simulink model "ev-obc-active-power-decoupling-model"  (R2025a)
settings: Solver=FixedStepAuto  StartTime=0.0  StopTime=1  FixedStep=1e-6  RelTol=1e-3
undefined symbols (not defined in the file): C_aux, k_current, k_power_alpha, k_power_beta, k_voltage, L_g, T_sw, Vbatt, w0
libraries: nesl_utility x12, fl_lib x11, ee_lib x4, spsAlphaBetaZerotodq0Lib x3, eeGeneralControl x2, slpidlib x2, spsdq0toAlphaBetaZeroLib x2
settings Model: Creator=AnasJ  LastModifiedBy=MEET

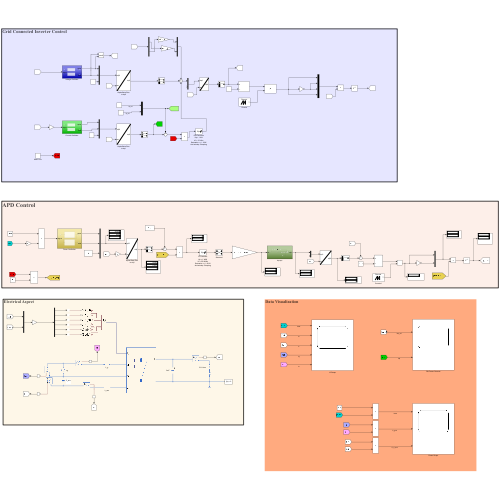
[thumbnail: Simulink's stored preview of the top-level diagram]
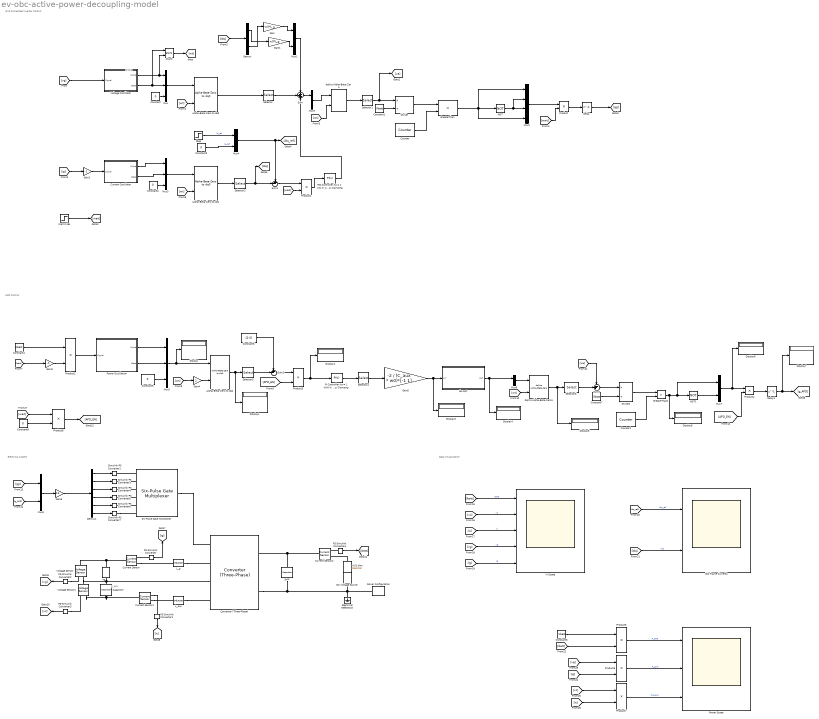
== system ev-obc-active-power-decoupling-model ==
  note: Data Visualization
  note: Electrical Aspect
  note: C_aux
  note: APD Control
  note: Grid Connected Inverter Control
  note: Alpha
  0.01 ohm : fl_lib/Electrical/Electrical Elements/Resistor  R=0.2 Ohm  i_specify=off  i_priority=None  i=0 A  i_nominal_specify=off  i_nominal_value=1  i_nominal_unit=A  v_specify=off  v_priority=None  v=0 V  v_nominal_specify=off  v_nominal_value=1  v_nominal_unit=V
  3mF : fl_lib/Electrical/Electrical Elements/Capacitor  c=3e-3 F  r=1e-6 Ohm  g=0 1/Ohm  i_specify=off  i_priority=None  i=0 A  i_nominal_specify=off  i_nominal_value=1  i_nominal_unit=A  v_specify=on  v_priority=High  v=400 V  v_nominal_specify=off  v_nominal_value=1  v_nominal_unit=V  vc_specify=off  vc_priority=High  vc=0 V  vc_nominal_specify=off  vc_nominal_value=1  vc_nominal_unit=V
  Alpha-Beta-Zero to dq0 : spsAlphaBetaZerotodq0Lib/Alpha-Beta-Zero to dq0  Alignment=90 degrees behind phase A axis
  Alpha-Beta-Zero to dq1 : spsAlphaBetaZerotodq0Lib/Alpha-Beta-Zero to dq0  Alignment=90 degrees behind phase A axis
  Alpha-Beta-Zero to dq2 : spsAlphaBetaZerotodq0Lib/Alpha-Beta-Zero to dq0  Alignment=90 degrees behind phase A axis
  Atan2 : Trigonometry  Operator=atan2
  Capacitor : fl_lib/Electrical/Electrical Elements/Capacitor  c=460 uF  r=1e-6 Ohm  g=0 1/Ohm  i_specify=off  i_priority=None  i=0 A  i_nominal_specify=off  i_nominal_value=1  i_nominal_unit=A  v_specify=off  v_priority=High  v=0 V  v_nominal_specify=off  v_nominal_value=1  v_nominal_unit=V  vc_specify=off  vc_priority=High  vc=0 V  vc_nominal_specify=off  vc_nominal_value=1  vc_nominal_unit=V
  Constant{,2..3,5,9} (5 alike) : Constant  Value=0
  Constant{1,4,7..8} (4 alike) : Constant  Value=Vbatt
  Constant6 : Constant  Value=[0 0]
  Converter (Three-Phase) : ee_lib/Semiconductors & Converters/Converters/Converter (Three-Phase)  port_option=ee.enum.threePhasePort.expanded  fidelity_option=ee.enum.converters.fidelity.detailed  device_type=ee.enum.converters.switchingdevice.ideal  showThermalPort=false  K=0  Vth=6 V  Vgt=1 V  Vgt_off=-1 V  Ih=1 A  Vf=0.8 V  Ron=0.001 Ohm  Rds=0.001 Ohm  Goff=1e-6 1/Ohm  Eon_scalar=22.86e-3 J  Eoff_scalar=17.14e-3 J  Eoff_natural_commutation=10e-3 J  Voff=300 V  Iout_scalar=600 A  onCurrentMeasDelay=0 s  useCurrentFromPreviousCycle=false  useVoltageFromPreviousCycle=false  diode_param=ee.enum.converters.protectiondiode.nodynamics  diode_Vf=0.8 V  diode_Ron=0.001 Ohm  diode_Goff=1e-5 1/Ohm  diode_C=50 nF  diode_iRM=-235 A  diode_iF=300 A  diode_idot=-50 A/us  diode_trr_param=ee.enum.converters.diodetrr.trr_factor  diode_trr_factor=3  diode_trr=15 us  diode_Qrr=1500 s*uA  diode_rec_loss_model=ee.enum.diode.reverseRecoveryModel.fixed  diode_ErecVal=0 J  diode_scaleWithIandV=false  diode_ErecMat=zeros(2, 3) J  diode_TjrecVec=[298.15, 398.15] K  diode_IfrecVec=[.1, 1, 10] A  diode_IrecVal=10 A  diode_VrecVal=10 V  diode_tFilter=1 / 1000 / 100 s  thermal_network_parameterization=ee.enum.thermalNetworkTopology.external  Rth=[.08, .5] K/W  Rth_Cauer=[.08, .1, .5] K/W  Rth_Foster=[.08, .14, .22, .16] K/W  thermal_mass_parameterization=ee.enum.thermalNetwork.timeconstant  thermal_mass=[.01, .5] J/K  thermal_mass_Cauer=[.01, .1, .5] J/K  thermal_mass_Foster=[.001, .005, .05, .5] J/K  thermal_time_constant=[.001, .2] s  thermal_time_constant_Cauer=[.001, .1, .2] s  thermal_time_constant_Foster=[7e-05, .0007, .01, .08] s  thermal_mass_initial_temperatures=[25, 25] degC  thermal_mass_initial_temperatures_Cauer=[25, 25, 25] degC  junction_thermal_mass=0.01 J/K  Tvec_initial_Foster=[25, 25, 25, 25] degC  snubber_type=ee.enum.converters.snubber.include  Cs=1e-7 F  Rs=0.1 Ohm  Vce_loss=[0, 150, 300] V
      settings: InternalSimscapePortConfiguration="{\"Bottom\":[],\"Left\":[{\"id\":\"G\",\"label\":\"G\",\"type\":\"foundation.electrical.twelve_phase\"},{\"id\":\"a\",\"label\":\"a\",\"type\":\"foundation.electrical.electrical\"},{\"id\":\"b\",\"label\":\"b\",\"type\":\"foundation.electrical.electrical\"},{\"id\":\"c\",\"label\":\"c\",\"type\":\"foundation.electrical.electrical\"}],\"Right\":[{\"id\":\"p\",\"label\":\"+\",\"type\":\"foundation.electrical.electrical\"},{\"id\":\"n\",\"label\":\"-\",\"type\":\"foundation.electrical.electrical\"}],\"Top\":[]}"
  Counter : eeGeneralControl/Counter  CarrCount=Up  Range=[0 1]  Tper=0.15  Tdelay=0  Ts=T_sw
      settings: LibrarySourceBlock=ee_sl_lib/General Control/Counter
  Counter1 : eeGeneralControl/Counter  CarrCount=Up  Range=[0 1]  Tper=0.15  Tdelay=0  Ts=T_sw
      settings: LibrarySourceBlock=ee_sl_lib/General Control/Counter
  Current Oscillator : Subsystem
  Current Sensor : fl_lib/Electrical/Electrical Sensors/Current Sensor
  Current Sensor1 : fl_lib/Electrical/Electrical Sensors/Current Sensor
  Current Sensor2 : fl_lib/Electrical/Electrical Sensors/Current Sensor
  DC Voltage Source : fl_lib/Electrical/Electrical Sources/DC Voltage Source  v0=400 V
  DQ Frame Currents : Scope  NumInputPorts=2
      settings: ActiveDisplayYMinimum=-56.25  ActiveDisplayYMaximum=6.2499999999999982
  Delay : Delay  DelayLength=1  InputProcessing=Columns as channels (frame based)
  Delay1 : Delay  DelayLength=1  InputProcessing=Columns as channels (frame based)
  Demux : Demux  Outputs=2
  Demux1 : Demux  Outputs=6
  Display{,1..8} (9 alike) : Display
  Divide : Product  Inputs=*/
  Divide1 : Product  Inputs=*/
  Electrical Reference : fl_lib/Electrical/Electrical Elements/Electrical Reference
  Gain : Gain  Gain=-w0*L_g
  Gain1 : Gain  Gain=w0*L_g
  Gain2 : Gain  Gain=-1
  Gain3 : Gain  Gain=-1
  Gain4 : Gain  Gain=2
  Gain5 : Gain  Gain=-2 / (C_aux * w0)*[-1 1]
  Gain6 : Gain  Gain=12
  GreaterThan : RelationalOperator  Operator=>  OutDataTypeStr=boolean  RndMeth=Simplest  InputSameDT=off
  GreaterThan1 : RelationalOperator  Operator=>  OutDataTypeStr=boolean  RndMeth=Simplest  InputSameDT=off
  L_aux : ee_lib/Passive/Inductor  l=55e-6 H  enable_L_tol=ee.enum.toleranceApplication.none  L_tol=20  tol_distribution=ee.enum.toleranceDistribution.uniform  nSigma=4  r=0.2 Ohm  g=1e-9 1/Ohm  enable_operating_limits=ee.enum.enable.no  operating_limit_action=ee.enum.passive.reportOpLim.warn  max_working_current=1 A  power_rating=1 W  i_L_specify=off  i_L_priority=High  i_L=0 A  i_L_nominal_specify=off  i_L_nominal_value=1  i_L_nominal_unit=A
  L_g : ee_lib/Passive/Inductor  l=16.35 mH  enable_L_tol=ee.enum.toleranceApplication.none  L_tol=20  tol_distribution=ee.enum.toleranceDistribution.uniform  nSigma=4  r=0.2 Ohm  g=1e-9 1/Ohm  enable_operating_limits=ee.enum.enable.no  operating_limit_action=ee.enum.passive.reportOpLim.warn  max_working_current=1 A  power_rating=1 W  i_L_specify=off  i_L_priority=High  i_L=0 A  i_L_nominal_specify=off  i_L_nominal_value=1  i_L_nominal_unit=A
  Mux : Mux  Inputs=3
  Mux{1,4,6..9} (6 alike) : Mux  Inputs=2
  Mux2 : Mux
  Mux3 : Mux  Inputs=3
  Mux5 : Mux  Inputs=3
  NOT : Logic  Operator=NOT  IconShape=distinctive  AllPortsSameDT=off  OutDataTypeStr=boolean
  NOT1 : Logic  Operator=NOT  IconShape=distinctive  AllPortsSameDT=off  OutDataTypeStr=boolean
  PI Controller Kp = 1 W/W Ki = 25 W/Ws Saturation = +/- 5e3V Anti-windup: Clamping : slpidlib/PID Controller  Controller=PI  Form=Parallel  TimeDomain=Continuous-time  UseExternalTs=off  SampleTime=-1  IntegratorMethod=Forward Euler  FilterMethod=Forward Euler  ControllerParametersSource=internal  P=1  I=25  UseKiTs=off  D=0  UseExternalDerivativeSource=off  N=100  UseFilter=on  TunerSelectOption=Transfer Function Based (PID Tuner App)  InitialConditionSource=internal  InitialConditionForIntegrator=0  InitialConditionForFilter=0  DifferentiatorICPrevScaledInput=0  ExternalReset=none  TrackingMode=off  Kt=1  LimitOutput=on  SatLimitsSource=internal  UpperSaturationLimit=5e3  LowerSaturationLimit=-5e3  LinearizeAsGain=on  AntiWindupMode=none  Kb=1  LimitIntegrator=off  UpperIntegratorSaturationLimit=inf  LowerIntegratorSaturationLimit=-inf  POutMin=[]  POutMax=[]  IOutMin=[]  IOutMax=[]  DOutMin=[]  DOutMax=[]  NOutMin=[]  NOutMax=[]  SumOutMin=[]  SumOutMax=[]  SaturationOutMin=[]  SaturationOutMax=[]  PParamMin=[]  PParamMax=[]  IParamMin=[]  IParamMax=[]  DParamMin=[]  DParamMax=[]  NParamMin=[]  NParamMax=[]  KbParamMin=[]  KbParamMax=[]  KtParamMin=[]  KtParamMax=[]  KbOutMin=[]  KbOutMax=[]  KtOutMin=[]  KtOutMax=[]  IntegratorOutMin=[]  IntegratorOutMax=[]  FilterOutMin=[]  FilterOutMax=[]  SumI1OutMin=[]  SumI1OutMax=[]  SumI2OutMin=[]  SumI2OutMax=[]  SumI3OutMin=[]  SumI3OutMax=[]  SumI4OutMin=[]  SumI4OutMax=[]  SumDOutMin=[]  SumDOutMax=[]  DifferentiatorOutMin=[]  DifferentiatorOutMax=[]  FilterDiffOutCoefMin=[]  FilterDiffOutCoefMax=[]  ReciprocalOutMin=[]  ReciprocalOutMax=[]  SumDenOutMin=[]  SumDenOutMax=[]  SumNumOutMin=[]  SumNumOutMax=[]  DivideOutMin=[]  DivideOutMax=[]  UdiffTsProdOutMin=[]  UdiffTsProdOutMax=[]  NTsProdOutMin=[]  NTsProdOutMax=[]  UintegralTsProdOutMin=[]  UintegralTsProdOutMax=[]  UngainTsProdOutMin=[]  UngainTsProdOutMax=[]  ClampingZeroOutDataTypeStr=Inherit: Inherit via back propagation  ClampingZeroOutMin=[]  ClampingZeroOutMax=[]  FilterDenConstantOutDataTypeStr=Inherit: Inherit via back propagation  FilterDenConstantOutMin=[]  FilterDenConstantOutMax=[]  PCopyOutDataTypeStr=Inherit: Inherit via back propagation  PCopyOutMin=[]  PCopyOutMax=[]  NCopyOutDataTypeStr=Inherit: Inherit via back propagation  NCopyOutMin=[]  NCopyOutMax=[]  IntegratorContinuousStateAttributes=''  IntegratorStateMustResolveToSignalObject=off  IntegratorRTWStateStorageClass=Auto  FilterContinuousStateAttributes=''  FilterStateMustResolveToSignalObject=off  FilterRTWStateStorageClass=Auto  ParallelPVariant=InternalParameters  IdealPVariant=Disabled  IVariant=InternalParameters  DVariant=Disabled  IntegratorVariant=Continuous  SatVariant=Enabled  AWVariant=Passthrough  PCopyVariant=Disabled  TRVariant=Disabled  FdbkBlocksVariant=Forward  IdealPFdbkVariant=Disabled  SatFdbkVariant=Disabled  DerivativeFilterVariant=Disabled  NVariant=Disabled  NCopyVariant=Disabled_SignalSpec  FilterICVariant=Disabled  IntegratorICVariant=InternalICs  ExternalResetVariant=Disabled  TRSumVariant=Passthrough  SumFdbkVariant=Disabled  SumVariant=Sum_PI  TsampFilterVariant=InternalTs  TsampNgainVariant=Passthrough  TsampIntegralVariant=Disabled_SignalSpec  ExternalSaturationOutDataTypeStr=Inherit: Same as second input  DerivativeSourceVariant=Disabled  PreIntVariant=InternalPreInt
  PID Controller Kp = 1 V/A Ki = 10 V/As Saturation = +/- 100V Anti-windup: Clamping : slpidlib/PID Controller  Controller=PI  Form=Parallel  TimeDomain=Continuous-time  UseExternalTs=off  SampleTime=-1  IntegratorMethod=Forward Euler  FilterMethod=Forward Euler  ControllerParametersSource=internal  P=5  I=50  UseKiTs=off  D=0  UseExternalDerivativeSource=off  N=100  UseFilter=on  TunerSelectOption=Transfer Function Based (PID Tuner App)  InitialConditionSource=internal  InitialConditionForIntegrator=0  InitialConditionForFilter=0  DifferentiatorICPrevScaledInput=0  ExternalReset=none  TrackingMode=off  Kt=1  LimitOutput=on  SatLimitsSource=internal  UpperSaturationLimit=100  LowerSaturationLimit=-100  LinearizeAsGain=on  AntiWindupMode=clamping  Kb=1  LimitIntegrator=off  UpperIntegratorSaturationLimit=inf  LowerIntegratorSaturationLimit=-inf  POutMin=[]  POutMax=[]  IOutMin=[]  IOutMax=[]  DOutMin=[]  DOutMax=[]  NOutMin=[]  NOutMax=[]  SumOutMin=[]  SumOutMax=[]  SaturationOutMin=[]  SaturationOutMax=[]  PParamMin=[]  PParamMax=[]  IParamMin=[]  IParamMax=[]  DParamMin=[]  DParamMax=[]  NParamMin=[]  NParamMax=[]  KbParamMin=[]  KbParamMax=[]  KtParamMin=[]  KtParamMax=[]  KbOutMin=[]  KbOutMax=[]  KtOutMin=[]  KtOutMax=[]  IntegratorOutMin=[]  IntegratorOutMax=[]  FilterOutMin=[]  FilterOutMax=[]  SumI1OutMin=[]  SumI1OutMax=[]  SumI2OutMin=[]  SumI2OutMax=[]  SumI3OutMin=[]  SumI3OutMax=[]  SumI4OutMin=[]  SumI4OutMax=[]  SumDOutMin=[]  SumDOutMax=[]  DifferentiatorOutMin=[]  DifferentiatorOutMax=[]  FilterDiffOutCoefMin=[]  FilterDiffOutCoefMax=[]  ReciprocalOutMin=[]  ReciprocalOutMax=[]  SumDenOutMin=[]  SumDenOutMax=[]  SumNumOutMin=[]  SumNumOutMax=[]  DivideOutMin=[]  DivideOutMax=[]  UdiffTsProdOutMin=[]  UdiffTsProdOutMax=[]  NTsProdOutMin=[]  NTsProdOutMax=[]  UintegralTsProdOutMin=[]  UintegralTsProdOutMax=[]  UngainTsProdOutMin=[]  UngainTsProdOutMax=[]  ClampingZeroOutDataTypeStr=Inherit: Inherit via back propagation  ClampingZeroOutMin=[]  ClampingZeroOutMax=[]  FilterDenConstantOutDataTypeStr=Inherit: Inherit via back propagation  FilterDenConstantOutMin=[]  FilterDenConstantOutMax=[]  PCopyOutDataTypeStr=Inherit: Inherit via back propagation  PCopyOutMin=[]  PCopyOutMax=[]  NCopyOutDataTypeStr=Inherit: Inherit via back propagation  NCopyOutMin=[]  NCopyOutMax=[]  IntegratorContinuousStateAttributes=''  IntegratorStateMustResolveToSignalObject=off  IntegratorRTWStateStorageClass=Auto  FilterContinuousStateAttributes=''  FilterStateMustResolveToSignalObject=off  FilterRTWStateStorageClass=Auto  ParallelPVariant=InternalParameters  IdealPVariant=Disabled  IVariant=InternalParameters  DVariant=Disabled  IntegratorVariant=Continuous  SatVariant=Enabled  AWVariant=ContClampingParallel  PCopyVariant=Disabled  TRVariant=Disabled  FdbkBlocksVariant=Forward  IdealPFdbkVariant=Disabled  SatFdbkVariant=Disabled  DerivativeFilterVariant=Disabled  NVariant=Disabled  NCopyVariant=Disabled_SignalSpec  FilterICVariant=Disabled  IntegratorICVariant=InternalICs  ExternalResetVariant=Disabled  TRSumVariant=Passthrough  SumFdbkVariant=Disabled  SumVariant=Sum_PI  TsampFilterVariant=InternalTs  TsampNgainVariant=Passthrough  TsampIntegralVariant=Disabled_SignalSpec  ExternalSaturationOutDataTypeStr=Inherit: Same as second input  DerivativeSourceVariant=Disabled  PreIntVariant=InternalPreInt
  PS-Simulink Converter{,1..4} (5 alike) : nesl_utility/PS-Simulink Converter  PhysicalDomain=network_engine_domain  SubClassName=ps_output  LeftPortType=input  RightPortType=output  PseudoPeriodic=off  Frequencies=[]  VectorFormat=inherit  Unit=inherit  AffineConversion=off
  Power Oscillation : Subsystem
  Power Scope : Scope  NumInputPorts=3
      settings: ActiveDisplayYMinimum=-891089.21436589747  ActiveDisplayYMaximum=99010.920853026575  DataLoggingVariableName=ScopeData2
  Product{,1..8} (9 alike) : Product
  Selector : Selector  InputPortWidth=3  IndexOptions=Index vector (dialog)  Indices=[1 2]  OutputSizes=1
  Selector1 : Selector  InputPortWidth=3  IndexOptions=Index vector (dialog)  Indices=[1]  OutputSizes=1
  Selector2 : Selector  InputPortWidth=3  IndexOptions=Index vector (dialog)  Indices=[1 2]  OutputSizes=1
  Selector3 : Selector  InputPortWidth=3  IndexOptions=Index vector (dialog)  Indices=[1 2]  OutputSizes=1
  Selector4 : Selector  InputPortWidth=2  IndexOptions=Index vector (dialog)  Indices=[2 1]  OutputSizes=1
  Selector5 : Selector  InputPortWidth=3  IndexOptions=Index vector (dialog)  Indices=[1]  OutputSizes=1
  Simulink-PS Converter{1,3..7} (6 alike) : nesl_utility/Simulink-PS Converter  PhysicalDomain=network_engine_domain  SubClassName=ps_input  LeftPortType=input  RightPortType=output  PseudoPeriodic=off  Frequencies=[]  NoiseDistribution=none  NoiseParameters=[]  Unit=1  AffineConversion=off  FilteringAndDerivatives=provide  SimscapeFilterOrder=1  InputFilterTimeConstant=0.001  UdotUserProvided=0
  Six-Pulse Gate Multiplexer : ee_lib/Semiconductors & Converters/Converters/Six-Pulse Gate Multiplexer  port_option=ee.enum.controlport.ps
  Solver Configuration : nesl_utility/Solver Configuration  PhysicalDomain=network_engine_domain  SubClassName=solver  LeftPortType=input  RightPortType=generic  Tones=[]  Harmonics=[]  SimulateNoise=off  Profile=off  UseLocalSampling=off  EnableSwitchedLinearOptims=on  FrequencyDomain=off  UseCCode=off  RelTol=0.001  AbsTol=0.001  MinStep=1e-09  ToWorkspace=off  RevertToSquareIcSolve=off  NumHomotopyIterations=100  PhasorMode=off  PhasorModeNumHarmonics=1  ConsistencySolver=NEWTON_XTOL_AFTER_FTOL  IndexReductionMethod=DerivativeReplacement  DoDC=off  ResidualTolerance=1e-09  ConsistencyTolSource=GLOBAL  ConsistencyAbsTol=0.001  ConsistencyRelTol=0.001  ConsistencyTolFactor=0.001  UseLocalSolver=on  LocalSolverChoice=NE_TRAPEZOIDAL_ADVANCER  ResolveIndetEquations=on  FunctionEvalNumThread=1  LocalSolverSampleTime=1e-6  DoFixedCost=off  MaxNonlinIter=3  MaxModeIter=2  ComputeImpulses=off  ImpulseIterations=2  LinearAlgebra=auto  LinearAlgebraNumThread=0  EquationFormulation=NE_TIME_EF  DelaysMemoryBudget=1024  AutomaticFiltering=on  FilteringTimeConstant=0.001  PartitionStorageMethod=AS_NEEDED  PartitionMemoryBudget=1024  PartitionMethod=ROBUST  MultibodyUseLocalSolver=off  MultibodyLocalSolverChoice=ODE1  MultibodyLocalSolverSampleTime=0.001
  Step : Step  Time=0.2  After=-50  SampleTime=0
  Sum : Sum  Inputs=+++
  Sum1 : Sum  Inputs=+-|
  Sum2 : Sum  Inputs=+-|
  Sum3 : Sum  Inputs=-+|
  VI Scope : Scope  NumInputPorts=5
      settings: ActiveDisplayYMinimum=-2227.7230359147438  ActiveDisplayYMaximum=247.52730213256646
  Voltage Oscillator : Subsystem
  Voltage Sensor : fl_lib/Electrical/Electrical Sensors/Voltage Sensor
  Voltage Sensor1 : fl_lib/Electrical/Electrical Sensors/Voltage Sensor
  Wait 0.15s : Step  Time=0.15  SampleTime=0
  dq-sqrt : Subsystem
  dq0 to Alpha-Beta-Zero : spsdq0toAlphaBetaZeroLib/dq0 to Alpha-Beta-Zero  Alignment=90 degrees behind phase A axis
  dq0 to Alpha-Beta-Zero1 : spsdq0toAlphaBetaZeroLib/dq0 to Alpha-Beta-Zero  Alignment=90 degrees behind phase A axis
  vg : fl_lib/Electrical/Electrical Sources/AC Voltage Source  amp=339.4 V  shift=0 deg  frequency=60 Hz
  wires:
  [vg] -> Voltage Oscillator/1(Signal)
  Constant/1 -> Mux/3
  Voltage Oscillator/2(Beta) -> Atan2/1, Mux/2
  Voltage Oscillator/1(Alpha) -> Atan2/2, Mux/1
  Atan2/1 -> [wt]
  Mux/1 -> Alpha-Beta-Zero to dq0/1
  [wt] -> Alpha-Beta-Zero to dq0/2
  Alpha-Beta-Zero to dq0/1 -> Selector/1
  [Idq] -> Demux/1
  Demux/2 -> Gain/1
  Demux/1 -> Gain1/1
  Selector/1 -> Sum/2
  Gain/1 -> Mux1/1
  Gain1/1 -> Mux1/2
  Mux1/1 -> Sum/1
  [wt] -> dq0 to Alpha-Beta-Zero/2
  dq0 to Alpha-Beta-Zero/1 -> Selector1/1
  Selector1/1 -> [va], Divide/1
  Constant1/1 -> Divide/2
  Divide/1 -> GreaterThan/1
  Counter/1 -> GreaterThan/2
  NOT/1 -> Mux2/3, Mux2/2
  GreaterThan/1 -> Mux2/4, Mux2/1, NOT/1
  Mux2/1 -> Product/1
  [wait] -> Product/2
  Product/1 -> Delay/1
  Delay/1 -> [gg]
  [ig] -> Gain2/1
  Wait 0.15s/1 -> [wait]
  Gain2/1 -> Current Oscillator/1(Signal)
  Current Oscillator/2(Beta) -> Mux3/2
  Current Oscillator/1(Alpha) -> Mux3/1
  Constant2/1 -> Mux3/3
  Mux3/1 -> Alpha-Beta-Zero to dq1/1
  [wt] -> Alpha-Beta-Zero to dq1/2
  Alpha-Beta-Zero to dq1/1 -> Selector2/1
  Constant3/1 -> Mux4/2  "Iq_ref"
  Step/1 -> Mux4/1  "Id_ref"
  Mux4/1 -> Sum1/1, [Idq_ref]
  Selector2/1 -> [Idq], Sum1/2
  Sum1/1 -> Product1/1
  [wait] -> Product1/2
  [ibatt] -> Gain3/1
  Gain3/1 -> Product2/2
  Constant4/1 -> Product2/1
  Product2/1 -> Power Oscillation/1(Signal)
  Power Oscillation/2(Beta) -> Mux5/2
  Power Oscillation/1(Alpha) -> Mux5/1
  Constant5/1 -> Mux5/3
  [wt] -> Gain4/1
  Gain4/1 -> Alpha-Beta-Zero to dq2/2
  Mux5/1 -> Display/1, Alpha-Beta-Zero to dq2/1
  Alpha-Beta-Zero to dq2/1 -> Display1/1, Selector3/1
  Selector3/1 -> Sum2/2
  Constant6/1 -> Sum2/1
  Sum2/1 -> Product3/1
  Product3/1 -> Display2/1, PI Controller Kp = 1 W/W Ki = 25 W/Ws Saturation = +/- 5e3V Anti-windup: Clamping/1
  PI Controller Kp = 1 W/W Ki = 25 W/Ws Saturation = +/- 5e3V Anti-windup: Clamping/1 -> Selector4/1
  Selector4/1 -> Gain5/1
  [wt] -> dq0 to Alpha-Beta-Zero1/2
  dq0 to Alpha-Beta-Zero1/1 -> Display5/1, Selector5/1
  Selector5/1 -> Sum3/2
  [va] -> Sum3/1
  Sum3/1 -> Divide1/1
  Constant7/1 -> Divide1/2
  Mux6/1 -> dq0 to Alpha-Beta-Zero1/1
  Divide1/1 -> GreaterThan1/1
  Counter1/1 -> GreaterThan1/2
  NOT1/1 -> Mux7/2
  GreaterThan1/1 -> Display6/1, NOT1/1, Mux7/1
  Mux7/1 -> Display8/1, Product4/1
  [APD_EN] -> Product4/2
  Product4/1 -> Delay1/1
  Delay1/1 -> Display7/1, [g_APD]
  [g_APD] -> Mux8/2
  [gg] -> Mux8/1
  Mux8/1 -> Gain6/1
  Demux1/1 -> Simulink-PS Converter1/1
  Demux1/2 -> Simulink-PS Converter3/1
  Demux1/3 -> Simulink-PS Converter4/1
  Gain6/1 -> Demux1/1
  Demux1/4 -> Simulink-PS Converter5/1
  Demux1/5 -> Simulink-PS Converter6/1
  Demux1/6 -> Simulink-PS Converter7/1
  PS-Simulink Converter/1 -> [ig]
  PS-Simulink Converter1/1 -> [ic]
  PS-Simulink Converter2/1 -> [vg]
  PS-Simulink Converter3/1 -> [vc]
  PS-Simulink Converter4/1 -> [ibatt]
  [ibatt] -> VI Scope/1  "Ibatt"
  [vc] -> VI Scope/2  "vc"
  [ic] -> VI Scope/3  "ic"
  [vg] -> VI Scope/4  "vg"
  [ig] -> VI Scope/5  "ig"
  [Idq_ref] -> DQ Frame Currents/1  "Idq_ref"
  [Idq] -> DQ Frame Currents/2  "Idq"
  Product7/1 -> Power Scope/3  "P_C_aux"
  Product6/1 -> Power Scope/2  "P_grid"
  Product5/1 -> Power Scope/1  "P_batt"
  Constant8/1 -> Product5/1
  [ibatt] -> Product5/2
  [vg] -> Product6/1
  [ig] -> Product6/2
  [vc] -> Product7/1
  [ic] -> Product7/2
  Sum/1 -> Mux9/1
  Mux9/1 -> dq0 to Alpha-Beta-Zero/1
  Constant9/1 -> Product8/2
  [wait] -> Product8/1
  Product8/1 -> [APD_EN]
  [APD_EN] -> Product3/2
  dq-sqrt/1(sqrt) -> Display4/1, Mux6/1
  Gain5/1 -> Display3/1, dq-sqrt/1(arr)
  Product1/1 -> PID Controller Kp = 1 V/A Ki = 10 V/As Saturation = +/- 100V Anti-windup: Clamping/1
  PID Controller Kp = 1 V/A Ki = 10 V/As Saturation = +/- 100V Anti-windup: Clamping/1 -> Sum/3
  connections:
  Six-Pulse Gate Multiplexer/LConn1 -- Simulink-PS Converter1/RConn1
  Simulink-PS Converter3/RConn1 -- Six-Pulse Gate Multiplexer/LConn2
  Simulink-PS Converter4/RConn1 -- Six-Pulse Gate Multiplexer/LConn3
  Simulink-PS Converter5/RConn1 -- Six-Pulse Gate Multiplexer/LConn4
  Simulink-PS Converter6/RConn1 -- Six-Pulse Gate Multiplexer/LConn5
  Simulink-PS Converter7/RConn1 -- Six-Pulse Gate Multiplexer/LConn6
  Six-Pulse Gate Multiplexer/RConn1 -- Converter (Three-Phase)/LConn1
  L_g/RConn1 -- Converter (Three-Phase)/LConn2
  L_aux/RConn1 -- Converter (Three-Phase)/LConn4
  Current Sensor/RConn2 -- L_g/LConn1
  PS-Simulink Converter/LConn1 -- Current Sensor/RConn1
  vg/LConn1 -- Current Sensor/LConn1 -- Voltage Sensor/LConn1
  Current Sensor1/RConn2 -- L_aux/LConn1
  Capacitor/RConn1 -- Current Sensor1/LConn1 -- Voltage Sensor1/RConn2
  Current Sensor1/RConn1 -- PS-Simulink Converter1/LConn1
  PS-Simulink Converter2/LConn1 -- Voltage Sensor/RConn1
  PS-Simulink Converter3/LConn1 -- Voltage Sensor1/RConn1
  Current Sensor2/LConn1 -- 3mF/LConn1 -- Converter (Three-Phase)/RConn1
  0.01 ohm/LConn1 -- Current Sensor2/RConn2
  DC Voltage Source/LConn1 -- 0.01 ohm/RConn1
  Converter (Three-Phase)/RConn2 -- 3mF/RConn1 -- Electrical Reference/LConn1 -- DC Voltage Source/RConn1 -- Solver Configuration/RConn1
  PS-Simulink Converter4/LConn1 -- Current Sensor2/RConn1
  Capacitor/LConn1 -- Voltage Sensor1/LConn1 -- Voltage Sensor/RConn2 -- vg/RConn1 -- Converter (Three-Phase)/LConn3

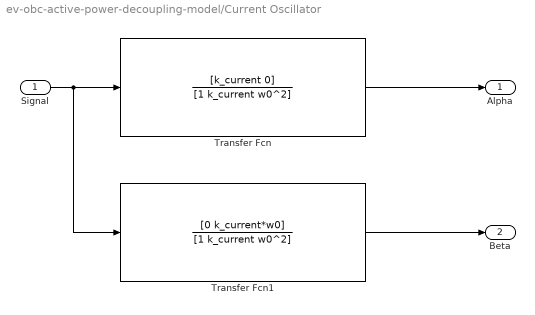
== system ev-obc-active-power-decoupling-model/Current Oscillator ==
  Signal : Inport
  Transfer Fcn : TransferFcn  Numerator=[k_current 0]  Denominator=[1 k_current w0^2]
  Transfer Fcn1 : TransferFcn  Numerator=[0 k_current*w0]  Denominator=[1 k_current w0^2]
  Alpha : Outport
  Beta : Outport  Port=2
  wires:
  Signal/1 -> Transfer Fcn1/1, Transfer Fcn/1
  Transfer Fcn/1 -> Alpha/1
  Transfer Fcn1/1 -> Beta/1

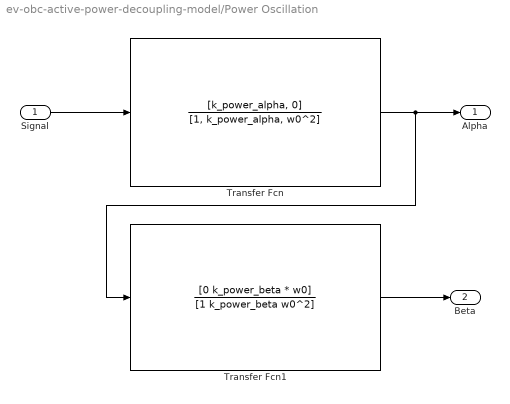
== system ev-obc-active-power-decoupling-model/Power Oscillation ==
  Signal : Inport
  Transfer Fcn : TransferFcn  Numerator=[k_power_alpha, 0]  Denominator=[1, k_power_alpha, w0^2]
  Transfer Fcn1 : TransferFcn  Numerator=[0 k_power_beta * w0]  Denominator=[1 k_power_beta w0^2]
  Alpha : Outport
  Beta : Outport  Port=2
  wires:
  Signal/1 -> Transfer Fcn/1
  Transfer Fcn/1 -> Transfer Fcn1/1, Alpha/1
  Transfer Fcn1/1 -> Beta/1

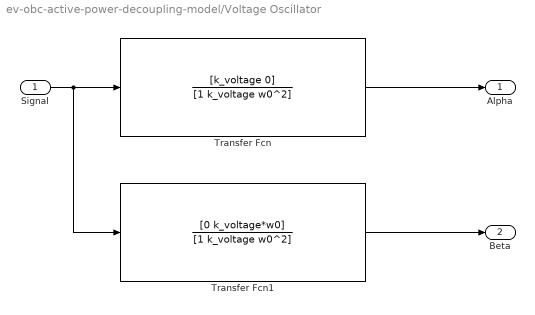
== system ev-obc-active-power-decoupling-model/Voltage Oscillator ==
  Signal : Inport
  Transfer Fcn : TransferFcn  Numerator=[k_voltage 0]  Denominator=[1 k_voltage w0^2]
  Transfer Fcn1 : TransferFcn  Numerator=[0 k_voltage*w0]  Denominator=[1 k_voltage w0^2]
  Alpha : Outport
  Beta : Outport  Port=2
  wires:
  Signal/1 -> Transfer Fcn1/1, Transfer Fcn/1
  Transfer Fcn/1 -> Alpha/1
  Transfer Fcn1/1 -> Beta/1

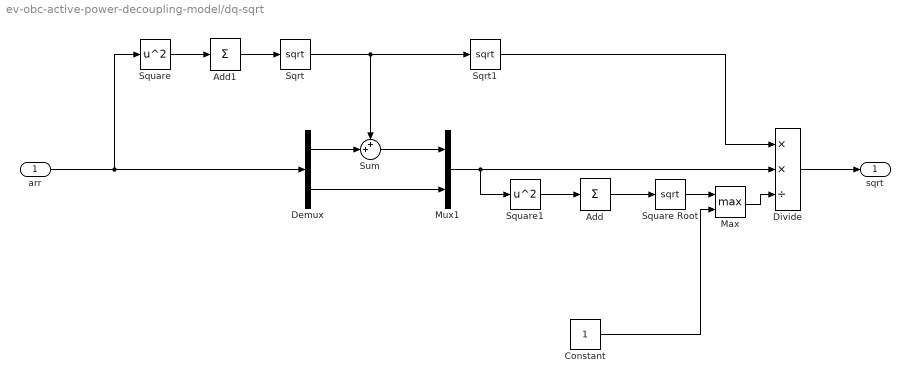
== system ev-obc-active-power-decoupling-model/dq-sqrt ==
  arr : Inport
  Add : Sum  Inputs=+
  Add1 : Sum  Inputs=+
  Constant : Constant
  Demux : Demux  Outputs=2
  Divide : Product  Inputs=**/
  Max : MinMax  Function=max  Inputs=2
  Mux1 : Mux  Inputs=2
  Sqrt : Sqrt
  Sqrt1 : Sqrt
  Square : Math  Operator=square
  Square Root : Sqrt
  Square1 : Math  Operator=square
  Sum : Sum  Inputs=++|
  sqrt : Outport
  wires:
  Square/1 -> Add1/1
  Add1/1 -> Sqrt/1
  Sqrt/1 -> Sqrt1/1, Sum/1
  Demux/1 -> Sum/2
  Sum/1 -> Mux1/1
  Demux/2 -> Mux1/2
  arr/1 -> Square/1, Demux/1
  Sqrt1/1 -> Divide/1
  Mux1/1 -> Square1/1, Divide/2
  Square1/1 -> Add/1
  Add/1 -> Square Root/1
  Divide/1 -> sqrt/1
  Square Root/1 -> Max/1
  Max/1 -> Divide/3
  Constant/1 -> Max/2
